simulink model "step6_2_setup_feedback_test"  (R2021b)
settings: Solver=ode45  StartTime=0.0  StopTime=15  RelTol=1e-3  EnableMultiTasking=on
values from neighbouring files (symbols this model uses):
  A = [0 1 0 0 ... (first row only)    [linearize_script.m]    (also in step4_0_linearize_operating_point.m = double(A); step4_linearized_system.mat = [0 0.339319496362 0 -114.426616159 0 1 -102.612245897 0 221.; syms_test.m = double(A))
  adingain = [adin_gain 1 1 1 1 1]    [hwinit.m]    (also in hwinit_raw.m)
  adinoffs = [adin_offs 0 0 0 0 0]    [hwinit.m]    (also in hwinit_raw.m)
  B = [0 ... (first row only)    [linearize_script.m]    (also in step4_0_linearize_operating_point.m = double(B); step4_linearized_system.mat = [0 0 0 0 5076.90787281]; syms_test.m = double(B))
  C = [1 0 0 0 ... (first row only)    [linearize_script.m]    (also in matrixmaker_linearization.m = [b_1_0 - P_3 * theta_d_2 * sin(theta_2)  -P_3 * (theta_d_1 +; step4_0_linearize_operating_point.m = [1 0 0 0 0; step4_linearized_system.mat = [1  0  0  0  0; 0  0  1  0  0]; syms_test.m)
  D = zeros(2,1)    [linearize_script.m]    (also in step4_0_linearize_operating_point.m; step4_linearized_system.mat = [0 0]; syms_test.m)
  daoutgain = 1*[-6]    [hwinit.m]    (also in hwinit_raw.m)
  daoutoffs = [0.00]    [hwinit.m]    (also in hwinit_raw.m)
  h = 0.001    [hwinit.m]    (also in hwinit_raw.m; init_fugi.m = fugiboard('Open', 'Pendulum1'); one_run.m = fugiboard('Open', 'pendulum1'); one_single_run.m = fugiboard('Open', 'pendulum1'))
  K = K1    [step6_1_controller_feedback.m]
  Ke = [165.387583111  -5.89857635124; 3165.93278733  -398.274578992; 81.102554045  215.74157361; 15046.5760039  11054.3649817; 3886.10400765  -704.144825536]    [step5_observor.mat]    (also in step5_observor_design.m = place(A_, B_, 0.5*J)')
  theta_1_0 = pi    (= 3.14159265359)    [hwinit.m]    (also in hwinit_raw.m; step4_0_linearize_operating_point.m; step5_observor_design.m = x_op(1); step6_1_controller_feedback.m = x_op(1))
  theta_2_0 = 0    [hwinit.m]    (also in hwinit_raw.m; step4_0_linearize_operating_point.m; step5_observor_design.m = x_op(3); step6_1_controller_feedback.m = x_op(3))
settings Model: Creator=rbabuska  LastModifiedBy=97083
settings SolverCC: AlgebraicLoopSolver=TrustRegion
settings DataIOCC: LimitDataPoints=on  SaveFormat=Array  ReturnWorkspaceOutputs=off  SignalLoggingName=sigsOut
settings OptimizationCC: BooleanDataType=off  ExpressionDepthLimit=2147483647  InitFltsAndDblsToZero=on  LifeSpan=inf
settings DebuggingCC: SaveWithParameterizedLinksMsg=none  SignalResolutionControl=TryResolveAllWithWarning  MultiTaskDSMMsg=warning  MultiTaskCondExecSysMsg=none  AllowSymbolicDim=off  StateNameClashWarn=warning  SFUnexpectedBacktrackingDiag=warning  SFNoUnconditionalDefaultTransitionDiag=warning  SFExecutionAtInitializationDiag=none  SFMachineParentedDataDiag=warning  ArithmeticOperatorsInVariantConditions=warning
settings HardwareCC: ProdBitPerPointer=32  ProdBitPerSizeT=32  ProdBitPerPtrDiffT=32  ProdLargestAtomicFloat=None  ProdIntDivRoundTo=Undefined  ProdEndianess=Unspecified  ProdWordSize=32  ProdHWDeviceType=32-bit Generic  TargetUnknown=on
settings ModelReferenceCC: PropagateSignalLabelsOutOfModel=off
settings SFSimCC: SimUseLocalCustomCode=off  CustomCodeUndefinedFunction=UseInterfaceOnly
settings RTWCC: RTWUseLocalCustomCode=off
settings CodeAppCC: StateflowObjectComments=on
settings GRTTargetCC: TargetFcnLib=ansi_tfl_tmw.mat  TargetLangStandard=C89/C90 (ANSI)  CombineOutputUpdateFcns=off  GRTInterface=on
settings ConfigComp: CovMetricSettings=dw  CovSaveCumulativeToWorkspaceVar=on  CovSaveSingleToWorkspaceVar=on  CovExternalEMLEnable=off

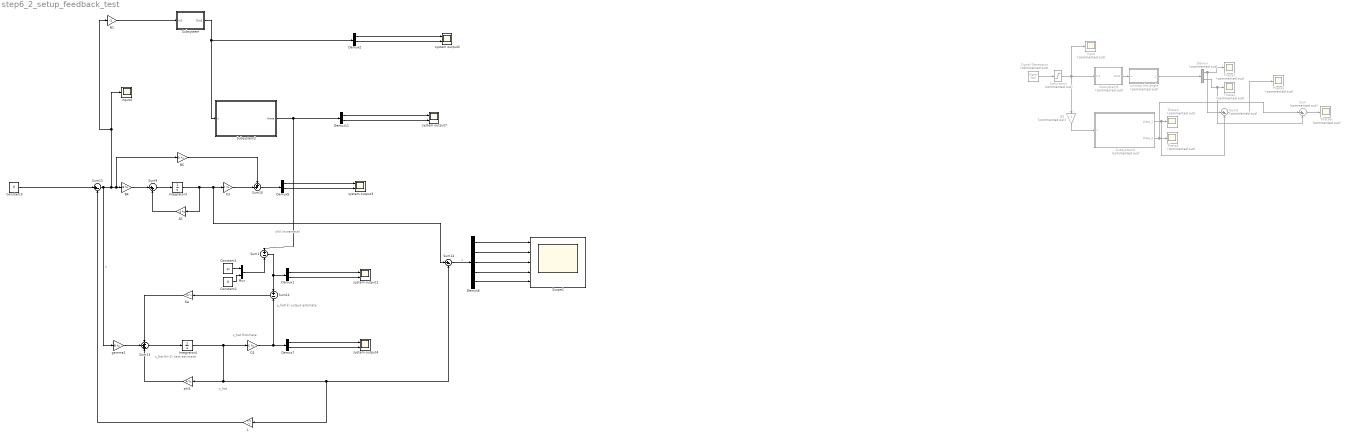
== system step6_2_setup_feedback_test ==
  note: y_hat(k)
      | output estimate
  note: x_hat(k+1)
      | next estimate
  note: y(k)
      | incremetal
  note: x_hat
      | Estimate
  note: x_hat
  A2 : Gain  Gain=A  Multiplication=Matrix(K*u) (u vector)
  B1 : Gain  Gain=-1
  B2 : Gain  Commented=on  Gain=-1
  B4 : Gain  Gain=B  Multiplication=Matrix(K*u)
  B5 : Gain  Gain=D  Multiplication=Matrix(K*u)
  C3 : Gain  Gain=C  Multiplication=Matrix(K*u) (u vector)
  C4 : Gain  Gain=C  Multiplication=Matrix(K*u) (u vector)
  Constant1 : Constant  Value=pi  SampleTime=-1
  Constant2 : Constant  Value=0  SampleTime=-1
  Constant3 : Constant  Value=0  SampleTime=0.001
  Demux : Demux  Commented=on  Outputs=2
  Demux{1..2,5,7,11} (5 alike) : Demux  Outputs=2
  Demux6 : Demux  Outputs=5
  Input : Scope  Commented=on
  Integrator3 : Integrator  InitialCondition=[0; 0; 0; 0; 0]
  Integrator4 : Integrator  InitialCondition=[0; 0; 0; 0; 0]
  Ke : Gain  Gain=Ke  Multiplication=Matrix(K*u) (u vector)
  L : Gain  Gain=1*K  Multiplication=Matrix(K*u) (u vector)
  Mux : Mux  Inputs=2
  Saturation : Saturate  Commented=on  UpperLimit=1  LowerLimit=-1
  Scope1 : Scope  NumInputPorts=5
  Signal Generator : SignalGenerator  Commented=on  Amplitude=0.5  Frequency=[1]
  Subsystem : Subsystem
      mask Display: disp('Rotational\nPendulum')
  Subsystem2 : Subsystem
  Subsystem4 : Subsystem  Commented=on
  Subsystem5 : Subsystem  Commented=on
      mask Display: disp('Rotational\nPendulum')
  Sum : Sum  Commented=on  Inputs=|+-
  Sum1 : Sum  Inputs=+|-
  Sum10 : Sum  Inputs=++|
  Sum11 : Sum  Inputs=|+-
  Sum12 : Sum  Inputs=+|-
  Sum13 : Sum  Inputs=+++
  Sum14 : Sum  Inputs=|+-
  Sum2 : Sum  Commented=on  Inputs=|+-
  Sum9 : Sum  Inputs=|++
  Theta{1..6} (6 alike) : Scope  Commented=on
  gamma1 : Gain  Gain=B  Multiplication=Matrix(K*u)
  input4 : Scope
  phi1 : Gain  Gain=A  Multiplication=Matrix(K*u) (u vector)
  system output{1..4,7} (5 alike) : Scope  NumInputPorts=2
  unwrap the angle : MATLAB Function  Commented=on  TreatAsAtomicUnit=on
  wires:
  Sum14/1 -> Demux6/1  "u"
  Constant3/1 -> Sum11/1
  Sum12/1 -> Ke/1
  Sum10/1 -> Demux5/1
  Integrator3/1 -> C3/1, Sum14/1, A2/1
  Sum9/1 -> Integrator3/1
  Demux7/1 -> system output4/1
  Demux5/2 -> system output3/2
  Ke/1 -> Sum13/1
  L/1 -> Sum11/2
  B4/1 -> Sum9/1
  phi1/1 -> Sum13/3
  Demux5/1 -> system output3/1
  Demux6/3 -> Scope1/3
  Demux7/2 -> system output4/2
  Demux6/5 -> Scope1/5
  B5/1 -> Sum10/1
  A2/1 -> Sum9/2
  Demux6/4 -> Scope1/4
  Sum13/1 -> Integrator4/1
  C4/1 -> Sum12/2, Demux7/1
  Demux11/2 -> system output7/2
  Demux6/1 -> Scope1/1
  Integrator4/1 -> phi1/1, L/1, Sum14/2, C4/1
  gamma1/1 -> Sum13/2
  Sum11/1 -> B1/1, input4/1, B4/1, B5/1, gamma1/1  "u"
  C3/1 -> Sum10/2
  Demux11/1 -> system output7/1
  Demux6/2 -> Scope1/2
  Sum1/1 -> Demux1/1, Sum12/1
  Constant1/1 -> Mux/1
  Constant2/1 -> Mux/2
  Demux1/1 -> system output1/1
  Demux1/2 -> system output1/2
  Mux/1 -> Sum1/2
  Subsystem2/1(theta) -> Sum1/1, Demux11/1
  Demux2/2 -> system output2/2
  Demux2/1 -> system output2/1
  Subsystem/1(Out1) -> Demux2/1, Subsystem2/1(u)
  B1/1 -> Subsystem/1(In1)
  Demux/1 -> Theta1/1, Sum2/1
  Subsystem5/1(Out1) -> unwrap the angle/1(u)
  Signal Generator/1 -> Saturation/1
  Saturation/1 -> B2/1, Subsystem5/1(In1), Input/1
  Subsystem4/1(theta_1) -> Sum2/2, Theta3/1
  Subsystem4/2(theta_2) -> Sum/1, Theta4/1
  B2/1 -> Subsystem4/1(u)
  unwrap the angle/1(y) -> Demux/1
  Demux/2 -> Sum/2, Theta2/1
  Sum2/1 -> Theta5/1
  Sum/1 -> Theta6/1

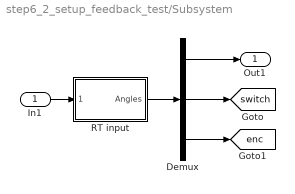
== system step6_2_setup_feedback_test/Subsystem ==
  In1 : Inport
  Demux : Demux  Outputs=[2 4 1]
  RT input : Subsystem  mask{Ts=h, channels=[6 7]}
      mask prompts: Ts "Sample time [s]:"; channels "Channels to read (e.g., [6 7])"
      mask init:
      | hwinit;
      | 
      | % initialize FPGA
      | fugihandle = fugiboard('Open', 'Pendulum1');
      | fugihandle.WatchdogTimeout = 0.5;
      | fugiboard('SetParams', fugihandle);
      | fugiboard('Write', fugihandle, 0, 0, 0, 0);  % dummy write to sync interface board
      | fugiboard('Write', fugihandle, 5, 1, 0, 0);  % reset position, activate relay
      | data = fugiboard('Read', fugihandle);        % get version info from FPGA
      | % model = bitshift(data(1), -5); 
      | % version = bitand(data(1), 31);
      | % disp(sprintf('FPGA setup %d, version %d', model, version)); % for the B&P it should say 1 1, or else there is a problem
      | fugiboard('Write', fugihandle, 0, 1, 0, 0);  % end reset
      | pause(0.1);                         % give relay some time to respond
      mask Display: disp('Rotational\nPendulum')
  Out1 : Outport
  tag scope: enc=global, switch=global
  wires:
  RT input/1(Angles) -> Demux/1
  Demux/1 -> Out1/1
  Demux/2 -> [switch]
  Demux/3 -> [enc]
  In1/1 -> RT input/1(Motors)

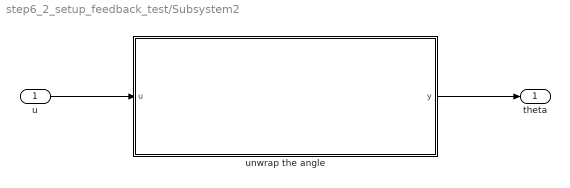
== system step6_2_setup_feedback_test/Subsystem2 ==
  u : Inport
  unwrap the angle : MATLAB Function  TreatAsAtomicUnit=on
  theta : Outport
  wires:
  u/1 -> unwrap the angle/1(u)
  unwrap the angle/1(y) -> theta/1

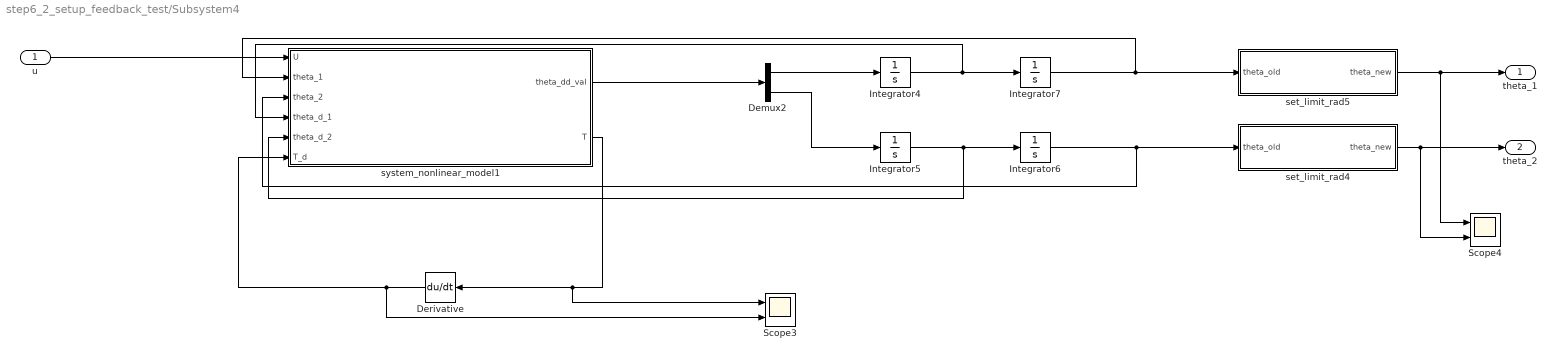
== system step6_2_setup_feedback_test/Subsystem4 ==
  u : Inport
  Demux2 : Demux  Outputs=2
  Derivative : Derivative  CoefficientInTFapproximation=0
  Integrator4 : Integrator
  Integrator5 : Integrator
  Integrator6 : Integrator  InitialCondition=theta_2_0
  Integrator7 : Integrator  InitialCondition=theta_1_0
  Scope3 : Scope  NumInputPorts=2
  Scope4 : Scope  NumInputPorts=2
  set_limit_rad4 : MATLAB Function  TreatAsAtomicUnit=on
  set_limit_rad5 : MATLAB Function  TreatAsAtomicUnit=on
  system_nonlinear_model1 : MATLAB Function  TreatAsAtomicUnit=on
  theta_1 : Outport
  theta_2 : Outport  Port=2
  wires:
  Derivative/1 -> Scope3/2, system_nonlinear_model1/6(T_d)
  system_nonlinear_model1/2(T) -> Scope3/1, Derivative/1
  set_limit_rad4/1(theta_new) -> theta_2/1, Scope4/2
  Integrator4/1 -> system_nonlinear_model1/4(theta_d_1), Integrator7/1
  system_nonlinear_model1/1(theta_dd_val) -> Demux2/1
  Integrator6/1 -> system_nonlinear_model1/3(theta_2), set_limit_rad4/1(theta_old)
  u/1 -> system_nonlinear_model1/1(U)
  Integrator7/1 -> set_limit_rad5/1(theta_old), system_nonlinear_model1/2(theta_1)
  Integrator5/1 -> system_nonlinear_model1/5(theta_d_2), Integrator6/1
  Demux2/1 -> Integrator4/1
  Demux2/2 -> Integrator5/1
  set_limit_rad5/1(theta_new) -> theta_1/1, Scope4/1

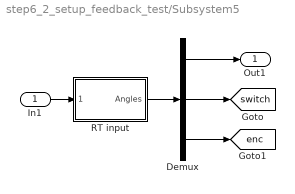
== system step6_2_setup_feedback_test/Subsystem5 ==
  In1 : Inport
  Demux : Demux  Outputs=[2 4 1]
  RT input : Subsystem  mask{Ts=h, channels=[6 7]}
      mask prompts: Ts "Sample time [s]:"; channels "Channels to read (e.g., [6 7])"
      mask init: same as step6_2_setup_feedback_test/Subsystem/RT input
      mask Display: disp('Rotational\nPendulum')
  Out1 : Outport
  tag scope: enc=global, switch=global
  wires:
  RT input/1(Angles) -> Demux/1
  Demux/1 -> Out1/1
  Demux/2 -> [switch]
  Demux/3 -> [enc]
  In1/1 -> RT input/1(Motors)

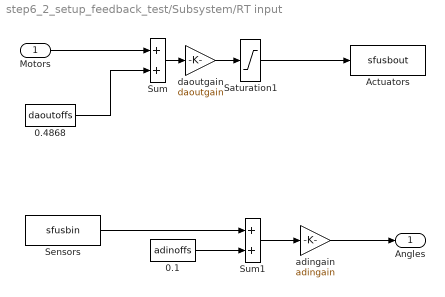
== system step6_2_setup_feedback_test/Subsystem/RT input ==
  Motors : Inport
  0.1 : Constant  Value=adinoffs
  0.4868 : Constant  Value=daoutoffs
  Actuators : S-Function  FunctionName=sfusbout  Parameters=Ts, fugihandle  SFunctionDeploymentMode=off  EnableBusSupport=off
  Saturation1 : Saturate  UpperLimit=10  LowerLimit=-10
  Sensors : S-Function  FunctionName=sfusbin  Parameters=Ts, fugihandle, channels  SFunctionDeploymentMode=off  EnableBusSupport=off
  Sum : Sum  InputSameDT=on  SaturateOnIntegerOverflow=on  OutDataTypeStr=Inherit: Same as first input
  Sum1 : Sum  InputSameDT=on  SaturateOnIntegerOverflow=on  OutDataTypeStr=Inherit: Same as first input
  adingain : Gain  Gain=adingain  SaturateOnIntegerOverflow=on  OutDataTypeStr=Inherit: Same as input  ParamDataTypeStr=Inherit: Same as input
  daoutgain : Gain  Gain=daoutgain  SaturateOnIntegerOverflow=on  OutDataTypeStr=Inherit: Same as input  ParamDataTypeStr=Inherit: Same as input
  Angles : Outport
  wires:
  Sum/1 -> daoutgain/1
  0.4868/1 -> Sum/2
  Motors/1 -> Sum/1
  Sum1/1 -> adingain/1
  0.1/1 -> Sum1/2
  adingain/1 -> Angles/1
  Saturation1/1 -> Actuators/1
  daoutgain/1 -> Saturation1/1
  Sensors/1 -> Sum1/1

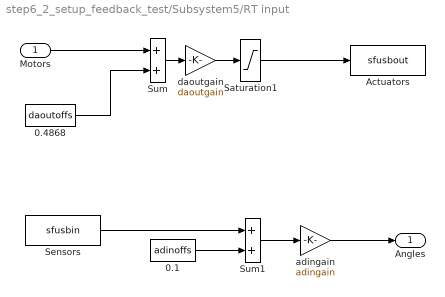
== system step6_2_setup_feedback_test/Subsystem5/RT input ==
  Motors : Inport
  0.1 : Constant  Value=adinoffs
  0.4868 : Constant  Value=daoutoffs
  Actuators : S-Function  FunctionName=sfusbout  Parameters=Ts, fugihandle  SFunctionDeploymentMode=off  EnableBusSupport=off
  Saturation1 : Saturate  UpperLimit=10  LowerLimit=-10
  Sensors : S-Function  FunctionName=sfusbin  Parameters=Ts, fugihandle, channels  SFunctionDeploymentMode=off  EnableBusSupport=off
  Sum : Sum  InputSameDT=on  SaturateOnIntegerOverflow=on  OutDataTypeStr=Inherit: Same as first input
  Sum1 : Sum  InputSameDT=on  SaturateOnIntegerOverflow=on  OutDataTypeStr=Inherit: Same as first input
  adingain : Gain  Gain=adingain  SaturateOnIntegerOverflow=on  OutDataTypeStr=Inherit: Same as input  ParamDataTypeStr=Inherit: Same as input
  daoutgain : Gain  Gain=daoutgain  SaturateOnIntegerOverflow=on  OutDataTypeStr=Inherit: Same as input  ParamDataTypeStr=Inherit: Same as input
  Angles : Outport
  wires:
  Sum/1 -> daoutgain/1
  0.4868/1 -> Sum/2
  Motors/1 -> Sum/1
  Sum1/1 -> adingain/1
  0.1/1 -> Sum1/2
  adingain/1 -> Angles/1
  Saturation1/1 -> Actuators/1
  daoutgain/1 -> Saturation1/1
  Sensors/1 -> Sum1/1

== matlab function step6_2_setup_feedback_test/Subsystem4/system_nonlinear_model1 ==
  settings: updateMethod=DISCRETE  sampleTime=0.001
  data: U input size=1; theta_dd_val output size=2; T output; theta_1 input size=1; theta_2 input size=1; theta_d_1 input size=1; theta_d_2 input size=1; T_d input
function [theta_dd_val, T]   = get_theta_dt_dt(U, theta_1, theta_2, theta_d_1, theta_d_2, T_d)


u = U(1);
k_m_0 = 65.9998023466922;
tau_e_0 = 0.003;
T = k_m_0 * u - tau_e_0 * T_d;

params = [-0.0300000121036330, 0.0203451968350115, 0.1000000000017210, 2.00882387117299e-05, 10.27570530021582, 0.78577414601457e-05, 49.9998023466922, 0.01500000000002200];  %found via white-box
% params = [-0.0984, 0.076, 0.074, 0.000045, 28.07, 0.000045, 25.9, 0.03];  %found via white-box
c_1_0 = params(1);
c_2_0 = params(2);
I_1_0 = params(3);
I_2_0 = params(4);
b_1_0 = params(5);
b_2_0 = params(6);





theta_dd_val = [
                                                                                                                                                                                                               theta_d_2*((200*b_2_0*(10*c_2_0^2 + cos(theta_2)*c_2_0 + 200*I_2_0))/(20*I_2_0 - c_2_0^2*cos(theta_2)^2 + 2000*I_1_0*c_2_0^2 + 5000*I_2_0*c_1_0^2 + c_2_0^2 + 250*c_1_0^2*c_2_0^2 + 40000*I_1_0*I_2_0) + (10*c_2_0*sin(theta_2)*(theta_d_1 + theta_d_2)*(c_2_0^2 + 20*I_2_0))/(20*I_2_0 - c_2_0^2*cos(theta_2)^2 + 2000*I_1_0*c_2_0^2 + 5000*I_2_0*c_1_0^2 + c_2_0^2 + 250*c_1_0^2*c_2_0^2 + 40000*I_1_0*I_2_0)) - theta_d_1*((2000*(c_2_0^2 + 20*I_2_0)*(b_1_0 - (c_2_0*theta_d_2*sin(theta_2))/200))/(20*I_2_0 - c_2_0^2*cos(theta_2)^2 + 2000*I_1_0*c_2_0^2 + 5000*I_2_0*c_1_0^2 + c_2_0^2 + 250*c_1_0^2*c_2_0^2 + 40000*I_1_0*I_2_0) - (c_2_0*theta_d_1*sin(theta_2)*(10*c_2_0^2 + cos(theta_2)*c_2_0 + 200*I_2_0))/(20*I_2_0 - c_2_0^2*cos(theta_2)^2 + 2000*I_1_0*c_2_0^2 + 5000*I_2_0*c_1_0^2 + c_2_0^2 + 250*c_1_0^2*c_2_0^2 + 40000*I_1_0*I_2_0)) + (2000*(sin(theta_1)*((981*c_1_0)/800 + 981/20000) + (981*c_2_0*sin(theta_1 + theta_2))/2000)*(c_2_0^2 + 20*I_2_0))/(20*I_2_0 - c_2_0^2*cos(theta_2)^2 + 2000*I_1_0*c_2_0^2 + 5000*I_2_0*c_1_0^2 + c_2_0^2 + 250*c_1_0^2*c_2_0^2 + 40000*I_1_0*I_2_0) + (2000*T*(c_2_0^2 + 20*I_2_0))/(20*I_2_0 - c_2_0^2*cos(theta_2)^2 + 2000*I_1_0*c_2_0^2 + 5000*I_2_0*c_1_0^2 + c_2_0^2 + 250*c_1_0^2*c_2_0^2 + 40000*I_1_0*I_2_0) - (981*c_2_0*sin(theta_1 + theta_2)*(10*c_2_0^2 + cos(theta_2)*c_2_0 + 200*I_2_0))/(10*(20*I_2_0 - c_2_0^2*cos(theta_2)^2 + 2000*I_1_0*c_2_0^2 + 5000*I_2_0*c_1_0^2 + c_2_0^2 + 250*c_1_0^2*c_2_0^2 + 40000*I_1_0*I_2_0))
theta_d_1*((200*(b_1_0 - (c_2_0*theta_d_2*sin(theta_2))/200)*(10*c_2_0^2 + cos(theta_2)*c_2_0 + 200*I_2_0))/(20*I_2_0 - c_2_0^2*cos(theta_2)^2 + 2000*I_1_0*c_2_0^2 + 5000*I_2_0*c_1_0^2 + c_2_0^2 + 250*c_1_0^2*c_2_0^2 + 40000*I_1_0*I_2_0) - (c_2_0*theta_d_1*sin(theta_2)*(250*c_1_0^2 + 100*c_2_0^2 + 20*cos(theta_2)*c_2_0 + 2000*I_1_0 + 2000*I_2_0 + 1))/(10*(20*I_2_0 - c_2_0^2*cos(theta_2)^2 + 2000*I_1_0*c_2_0^2 + 5000*I_2_0*c_1_0^2 + c_2_0^2 + 250*c_1_0^2*c_2_0^2 + 40000*I_1_0*I_2_0))) - theta_d_2*((20*b_2_0*(250*c_1_0^2 + 100*c_2_0^2 + 20*cos(theta_2)*c_2_0 + 2000*I_1_0 + 2000*I_2_0 + 1))/(20*I_2_0 - c_2_0^2*cos(theta_2)^2 + 2000*I_1_0*c_2_0^2 + 5000*I_2_0*c_1_0^2 + c_2_0^2 + 250*c_1_0^2*c_2_0^2 + 40000*I_1_0*I_2_0) + (c_2_0*sin(theta_2)*(theta_d_1 + theta_d_2)*(10*c_2_0^2 + cos(theta_2)*c_2_0 + 200*I_2_0))/(20*I_2_0 - c_2_0^2*cos(theta_2)^2 + 2000*I_1_0*c_2_0^2 + 5000*I_2_0*c_1_0^2 + c_2_0^2 + 250*c_1_0^2*c_2_0^2 + 40000*I_1_0*I_2_0)) - (200*(sin(theta_1)*((981*c_1_0)/800 + 981/20000) + (981*c_2_0*sin(theta_1 + theta_2))/2000)*(10*c_2_0^2 + cos(theta_2)*c_2_0 + 200*I_2_0))/(20*I_2_0 - c_2_0^2*cos(theta_2)^2 + 2000*I_1_0*c_2_0^2 + 5000*I_2_0*c_1_0^2 + c_2_0^2 + 250*c_1_0^2*c_2_0^2 + 40000*I_1_0*I_2_0) - (200*T*(10*c_2_0^2 + cos(theta_2)*c_2_0 + 200*I_2_0))/(20*I_2_0 - c_2_0^2*cos(theta_2)^2 + 2000*I_1_0*c_2_0^2 + 5000*I_2_0*c_1_0^2 + c_2_0^2 + 250*c_1_0^2*c_2_0^2 + 40000*I_1_0*I_2_0) + (981*c_2_0*sin(theta_1 + theta_2)*(250*c_1_0^2 + 100*c_2_0^2 + 20*cos(theta_2)*c_2_0 + 2000*I_1_0 + 2000*I_2_0 + 1))/(100*(20*I_2_0 - c_2_0^2*cos(theta_2)^2 + 2000*I_1_0*c_2_0^2 + 5000*I_2_0*c_1_0^2 + c_2_0^2 + 250*c_1_0^2*c_2_0^2 + 40000*I_1_0*I_2_0));
];

== matlab function step6_2_setup_feedback_test/unwrap the angle ==
  settings: updateMethod=DISCRETE  sampleTime=0.001
  data: u input size=2; y output size=2
function y = unwrap_angle(u)

y = unwrap(u);
y = u;

== matlab function step6_2_setup_feedback_test/Subsystem4/set_limit_rad4 ==
  settings: updateMethod=DISCRETE  sampleTime=0.001
  data: theta_old input size=1; theta_new output size=1
function theta_new   = set_limit_rad(theta_old)

% theta_new = theta_old - floor(theta_old / 2 / pi) * 2 * pi;
theta_new = theta_old;

== matlab function step6_2_setup_feedback_test/Subsystem4/set_limit_rad5 ==
  settings: updateMethod=DISCRETE  sampleTime=0.001
  data: theta_old input size=1; theta_new output size=1
function theta_new   = set_limit_rad(theta_old)

% theta_new = theta_old - floor(theta_old / 2 / pi) * 2 * pi;
theta_new = theta_old;

== matlab function step6_2_setup_feedback_test/Subsystem2/unwrap the angle ==
  settings: updateMethod=DISCRETE  sampleTime=0.001
  data: u input size=2; y output size=2
function y = unwrap_angle(u)

y = unwrap(u);
% y = u;
